simulink model "Sub_Gear"  (R2014a)
settings: Solver=ode45  StartTime=0.0  StopTime=10.0  RelTol=1e-3
undefined symbols (not defined in the file): K
settings Model: Creator=hsinwang  LastModifiedBy=hsinwang

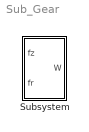
== system Sub_Gear ==
  Subsystem : Subsystem

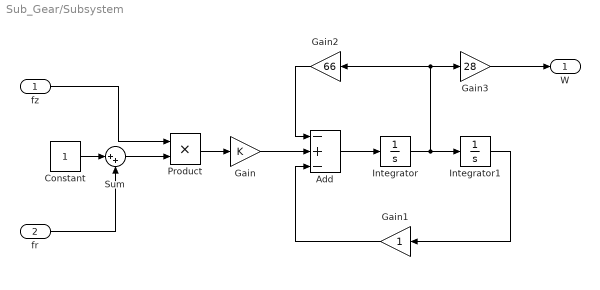
== system Sub_Gear/Subsystem ==
  "fz " : Inport
  "fr " : Inport  Port=2
  Add : Sum  Inputs=-+-
  Constant : Constant
  Gain : Gain  Gain=K
  Gain1 : Gain
  Gain2 : Gain  Gain=66
  Gain3 : Gain  Gain=28
  Integrator : Integrator
  Integrator1 : Integrator
  Product : Product
  Sum : Sum  Inputs=|++
  W : Outport
  wires:
  Constant/1 -> Sum/1
  "fr "/1 -> Sum/2
  Sum/1 -> Product/2
  "fz "/1 -> Product/1
  Product/1 -> Gain/1
  Gain/1 -> Add/2
  Add/1 -> Integrator/1
  Integrator/1 -> Integrator1/1, Gain3/1, Gain2/1
  Integrator1/1 -> Gain1/1
  Gain1/1 -> Add/3
  Gain2/1 -> Add/1
  Gain3/1 -> W/1
